simulink model "Modelo"  (R2018a)
settings: Solver=ode45  StartTime=0.0  StopTime=27  FixedStep=0.0001  MaxStep=1e-3
values from neighbouring files (symbols this model uses):
  d = 0.01    [setupSimulinkConstantes.m]
  erroInviavel_rotacao = pi    (= 3.14159265359)    [setupSimulinkConstantes.m]
  erroInviavel_translacao = 10    [setupSimulinkConstantes.m]
  J = 0.0015    [setupSimulinkConstantes.m]
  Kb = 0.4    [setupSimulinkConstantes.m]
  Kc = 4    [setupSimulinkConstantes.m]
  Kd = solucao(3)    [setupSimulinkSolucao.m]
  Ki = solucao(2)    [setupSimulinkSolucao.m]
  Kp = solucao(1)    [setupSimulinkSolucao.m]
  Kt = 0.4    [setupSimulinkConstantes.m]
  L = 0.1    [setupSimulinkConstantes.m]
  M = 0.25    [setupSimulinkConstantes.m]
  N = length(Xinit)    [Calcula_Delta_E.m]    (also in setupSimulinkConstantes.m = 30)
  Pista = 0    [ValidaResultado.m]    (also in fcusto_completa.m = i; fcusto_simplificada.m)
  R = 0.05    [setupSimulinkConstantes.m]
  Ra = 5e-3    (= 0.005)    [setupSimulinkConstantes.m]
  Va_med = 2.5    [setupSimulinkConstantes.m]
undefined symbols (not defined in the file or in its folder): sigbuilder_block
libraries: simulink x4
settings Model: SimulationMode=accelerator  Creator=root  LastModifiedBy=gabri
settings SolverCC: MaxConsecutiveZCs=100000  MaxConsecutiveMinStep=20
settings DataIOCC: ReturnWorkspaceOutputs=on
settings DebuggingCC: MaxConsecutiveZCsMsg=none  LibraryContextMissingDiagnostic=warning
settings SFSimCC: SimUseLocalCustomCode=on
settings RTWCC: RTWUseLocalCustomCode=on

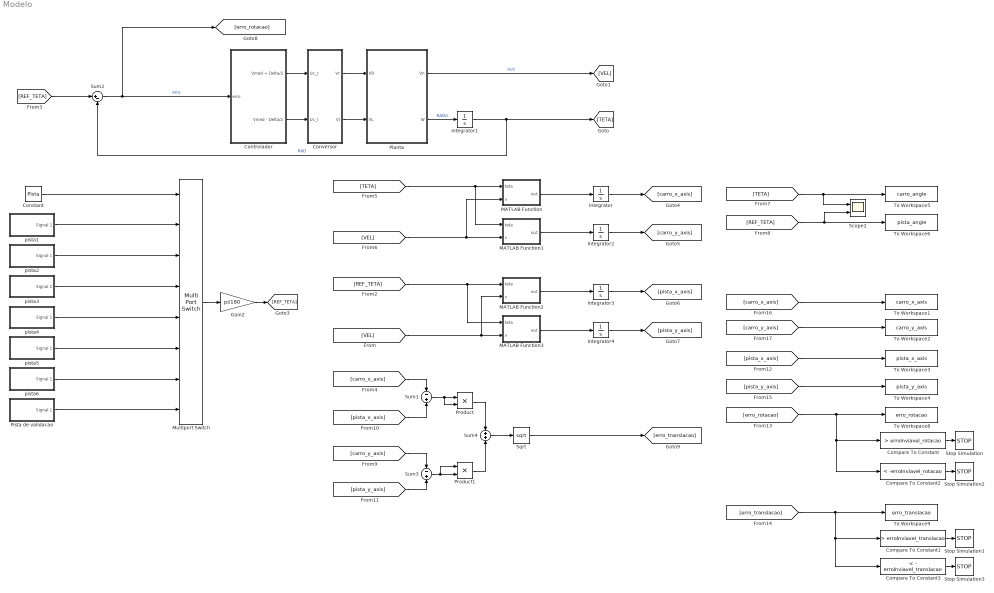
== system Modelo ==
  Compare To Constant : simulink/Logic and Bit Operations/Compare To Constant  relop=>  const=erroInviavel_rotacao  OutDataTypeStr=boolean
  Compare To Constant1 : simulink/Logic and Bit Operations/Compare To Constant  relop=>  const=erroInviavel_translacao  OutDataTypeStr=boolean
  Compare To Constant2 : simulink/Logic and Bit Operations/Compare To Constant  relop=<  const=-erroInviavel_rotacao  OutDataTypeStr=boolean
  Compare To Constant3 : simulink/Logic and Bit Operations/Compare To Constant  relop=<  const=- erroInviavel_translacao  OutDataTypeStr=boolean
  Constant : Constant  Value=Pista  VectorParams1D=off
  Controlador : Subsystem
  Conversor : Subsystem
  Gain2 : Gain  Gain=pi/180
  Integrator{,1..4} (5 alike) : Integrator
  MATLAB Function : MATLAB Function  TreatAsAtomicUnit=on
  MATLAB Function1 : MATLAB Function  TreatAsAtomicUnit=on
  MATLAB Function2 : MATLAB Function  TreatAsAtomicUnit=on
  MATLAB Function3 : MATLAB Function  TreatAsAtomicUnit=on
  Multiport Switch : MultiPortSwitch  Inputs=7  DiagnosticForDefault=None
  Pista de validacao : Subsystem  Tag=STV Subsys  LoadFcn=sigbuilder_block('load');  StartFcn=sigbuilder_block('start');  StopFcn=sigbuilder_block('stop');  ClipboardFcn=sigbuilder_block('clipboard');  mask(Sigbuilder block){tuvar=[0:10]}
      mask help: Simulink:masks:SigbuilderBlock_MD
      mask init:
      | if ~strcmp(get_param(bdroot(gcbh),'SimulationStatus'),'stopped') tuvar = sigbuilder_block('maskInit'); end
      settings: CopyFcn=sigbuilder_block('copy');  DeleteFcn=sigbuilder_block('delete');  ModelCloseFcn=sigbuilder_block('modelClose');  PreSaveFcn=sigbuilder_block('preSave');  PauseFcn=sigbuilder_block('pause');  ContinueFcn=sigbuilder_block('continue');  NameChangeFcn=sigbuilder_block('namechange');  OpenFcn=sigbuilder_block('open',[422.25 122.25 580.5 337.5 ]);  CloseFcn=sigbuilder_block('close');
      mask Display: plot(0, 0, 100, 100,[2, 2, 32, 32, 2], [68, 8, 8, 68, 68],[32, 2], [38, 38], [32, 19, 2],[53, 60, 44], [32, 17, 17, 2],[16, 16, 31, 31]);txt = getActiveGroup(gcbh);text(2, 100, txt,'verticalAlignment', 'top');
  Planta : Subsystem
  Product : Product
  Product1 : Product
  Scope2 : Scope  NumInputPorts=2
  Sqrt : Sqrt  SaturateOnIntegerOverflow=on
  Stop Simulation{,1..3} (4 alike) : Stop
  Sum1 : Sum  Inputs=-|+
  Sum2 : Sum  Inputs=|+-
  Sum3 : Sum  Inputs=-|+
  Sum4 : Sum  Inputs=+|+
  To Workspace1 : ToWorkspace  VariableName=carro_x_axis  SampleTime=-1
      settings: Save2DSignal=2-D array (concatenate along first dimension)
  To Workspace2 : ToWorkspace  VariableName=carro_y_axis  SampleTime=-1
      settings: Save2DSignal=2-D array (concatenate along first dimension)
  To Workspace3 : ToWorkspace  VariableName=pista_x_axis  SampleTime=-1
      settings: Save2DSignal=2-D array (concatenate along first dimension)
  To Workspace4 : ToWorkspace  VariableName=pista_y_axis  SampleTime=-1
      settings: Save2DSignal=2-D array (concatenate along first dimension)
  To Workspace5 : ToWorkspace  VariableName=carro_angle  SampleTime=-1
      settings: Save2DSignal=2-D array (concatenate along first dimension)
  To Workspace6 : ToWorkspace  VariableName=pista_angle  SampleTime=-1
      settings: Save2DSignal=2-D array (concatenate along first dimension)
  To Workspace8 : ToWorkspace  VariableName=erro_rotacao  SampleTime=-1
      settings: Save2DSignal=2-D array (concatenate along first dimension)
  To Workspace9 : ToWorkspace  VariableName=erro_translacao  SampleTime=-1
      settings: Save2DSignal=2-D array (concatenate along first dimension)
  pista1 : Subsystem  Tag=STV Subsys  LoadFcn=sigbuilder_block('load');  StartFcn=sigbuilder_block('start');  StopFcn=sigbuilder_block('stop');  ClipboardFcn=sigbuilder_block('clipboard');  mask(Sigbuilder block){tuvar=[0:10]}
      mask help: Simulink:masks:SigbuilderBlock_MD
      mask init:
      | if ~strcmp(get_param(bdroot(gcbh),'SimulationStatus'),'stopped') tuvar = sigbuilder_block('maskInit'); end
      settings: CopyFcn=sigbuilder_block('copy');  DeleteFcn=sigbuilder_block('delete');  ModelCloseFcn=sigbuilder_block('modelClose');  PreSaveFcn=sigbuilder_block('preSave');  PauseFcn=sigbuilder_block('pause');  ContinueFcn=sigbuilder_block('continue');  NameChangeFcn=sigbuilder_block('namechange');  OpenFcn=sigbuilder_block('open',[426 126 573 342.75 ]);  CloseFcn=sigbuilder_block('close');
      mask Display: plot(0, 0, 100, 100,[2, 2, 32, 32, 2], [68, 8, 8, 68, 68],[32, 2], [38, 38], [32, 19, 2],[53, 60, 44], [32, 17, 17, 2],[16, 16, 31, 31]);txt = getActiveGroup(gcbh);text(2, 100, txt,'verticalAlignment', 'top');
  pista2 : Subsystem  Tag=STV Subsys  LoadFcn=sigbuilder_block('load');  StartFcn=sigbuilder_block('start');  StopFcn=sigbuilder_block('stop');  ClipboardFcn=sigbuilder_block('clipboard');  mask(Sigbuilder block){tuvar=[0:10]}
      mask help: Simulink:masks:SigbuilderBlock_MD
      mask init:
      | if ~strcmp(get_param(bdroot(gcbh),'SimulationStatus'),'stopped') tuvar = sigbuilder_block('maskInit'); end
      settings: CopyFcn=sigbuilder_block('copy');  DeleteFcn=sigbuilder_block('delete');  ModelCloseFcn=sigbuilder_block('modelClose');  PreSaveFcn=sigbuilder_block('preSave');  PauseFcn=sigbuilder_block('pause');  ContinueFcn=sigbuilder_block('continue');  NameChangeFcn=sigbuilder_block('namechange');  OpenFcn=sigbuilder_block('open',[403.5 98.25 610.5 316.5 ]);  CloseFcn=sigbuilder_block('close');
      mask Display: plot(0, 0, 100, 100,[2, 2, 32, 32, 2], [68, 8, 8, 68, 68],[32, 2], [38, 38], [32, 19, 2],[53, 60, 44], [32, 17, 17, 2],[16, 16, 31, 31]);txt = getActiveGroup(gcbh);text(2, 100, txt,'verticalAlignment', 'top');
  pista3 : Subsystem  Tag=STV Subsys  LoadFcn=sigbuilder_block('load');  StartFcn=sigbuilder_block('start');  StopFcn=sigbuilder_block('stop');  ClipboardFcn=sigbuilder_block('clipboard');  mask(Sigbuilder block){tuvar=[0:10]}
      mask help: Simulink:masks:SigbuilderBlock_MD
      mask init:
      | if ~strcmp(get_param(bdroot(gcbh),'SimulationStatus'),'stopped') tuvar = sigbuilder_block('maskInit'); end
      settings: CopyFcn=sigbuilder_block('copy');  DeleteFcn=sigbuilder_block('delete');  ModelCloseFcn=sigbuilder_block('modelClose');  PreSaveFcn=sigbuilder_block('preSave');  PauseFcn=sigbuilder_block('pause');  ContinueFcn=sigbuilder_block('continue');  NameChangeFcn=sigbuilder_block('namechange');  OpenFcn=sigbuilder_block('open',[407.25 107.25 610.5 316.5 ]);  CloseFcn=sigbuilder_block('close');
      mask Display: plot(0, 0, 100, 100,[2, 2, 32, 32, 2], [68, 8, 8, 68, 68],[32, 2], [38, 38], [32, 19, 2],[53, 60, 44], [32, 17, 17, 2],[16, 16, 31, 31]);txt = getActiveGroup(gcbh);text(2, 100, txt,'verticalAlignment', 'top');
  pista4 : Subsystem  Tag=STV Subsys  LoadFcn=sigbuilder_block('load');  StartFcn=sigbuilder_block('start');  StopFcn=sigbuilder_block('stop');  ClipboardFcn=sigbuilder_block('clipboard');  mask(Sigbuilder block){tuvar=[0:10]}
      mask help: Simulink:masks:SigbuilderBlock_MD
      mask init:
      | if ~strcmp(get_param(bdroot(gcbh),'SimulationStatus'),'stopped') tuvar = sigbuilder_block('maskInit'); end
      settings: CopyFcn=sigbuilder_block('copy');  DeleteFcn=sigbuilder_block('delete');  ModelCloseFcn=sigbuilder_block('modelClose');  PreSaveFcn=sigbuilder_block('preSave');  PauseFcn=sigbuilder_block('pause');  ContinueFcn=sigbuilder_block('continue');  NameChangeFcn=sigbuilder_block('namechange');  OpenFcn=sigbuilder_block('open',[422.25 122.25 580.5 337.5 ]);  CloseFcn=sigbuilder_block('close');
      mask Display: plot(0, 0, 100, 100,[2, 2, 32, 32, 2], [68, 8, 8, 68, 68],[32, 2], [38, 38], [32, 19, 2],[53, 60, 44], [32, 17, 17, 2],[16, 16, 31, 31]);txt = getActiveGroup(gcbh);text(2, 100, txt,'verticalAlignment', 'top');
  pista5 : Subsystem  Tag=STV Subsys  LoadFcn=sigbuilder_block('load');  StartFcn=sigbuilder_block('start');  StopFcn=sigbuilder_block('stop');  ClipboardFcn=sigbuilder_block('clipboard');  mask(Sigbuilder block){tuvar=[0:10]}
      mask help: Simulink:masks:SigbuilderBlock_MD
      mask init:
      | if ~strcmp(get_param(bdroot(gcbh),'SimulationStatus'),'stopped') tuvar = sigbuilder_block('maskInit'); end
      settings: CopyFcn=sigbuilder_block('copy');  DeleteFcn=sigbuilder_block('delete');  ModelCloseFcn=sigbuilder_block('modelClose');  PreSaveFcn=sigbuilder_block('preSave');  PauseFcn=sigbuilder_block('pause');  ContinueFcn=sigbuilder_block('continue');  NameChangeFcn=sigbuilder_block('namechange');  OpenFcn=sigbuilder_block('open',[411 100.5 588 332.25 ]);  CloseFcn=sigbuilder_block('close');
      mask Display: plot(0, 0, 100, 100,[2, 2, 32, 32, 2], [68, 8, 8, 68, 68],[32, 2], [38, 38], [32, 19, 2],[53, 60, 44], [32, 17, 17, 2],[16, 16, 31, 31]);txt = getActiveGroup(gcbh);text(2, 100, txt,'verticalAlignment', 'top');
  pista6 : Subsystem  Tag=STV Subsys  LoadFcn=sigbuilder_block('load');  StartFcn=sigbuilder_block('start');  StopFcn=sigbuilder_block('stop');  ClipboardFcn=sigbuilder_block('clipboard');  mask(Sigbuilder block){tuvar=[0:10]}
      mask help: Simulink:masks:SigbuilderBlock_MD
      mask init:
      | if ~strcmp(get_param(bdroot(gcbh),'SimulationStatus'),'stopped') tuvar = sigbuilder_block('maskInit'); end
      settings: CopyFcn=sigbuilder_block('copy');  DeleteFcn=sigbuilder_block('delete');  ModelCloseFcn=sigbuilder_block('modelClose');  PreSaveFcn=sigbuilder_block('preSave');  PauseFcn=sigbuilder_block('pause');  ContinueFcn=sigbuilder_block('continue');  NameChangeFcn=sigbuilder_block('namechange');  OpenFcn=sigbuilder_block('open',[414.75 114.75 595.5 327 ]);  CloseFcn=sigbuilder_block('close');
      mask Display: plot(0, 0, 100, 100,[2, 2, 32, 32, 2], [68, 8, 8, 68, 68],[32, 2], [38, 38], [32, 19, 2],[53, 60, 44], [32, 17, 17, 2],[16, 16, 31, 31]);txt = getActiveGroup(gcbh);text(2, 100, txt,'verticalAlignment', 'top');
  wires:
  Sum2/1 -> Controlador/1(erro), [erro_rotacao]  "erro"
  Integrator1/1 -> Sum2/2, [TETA]  "RAD"
  Planta/1(Vn) -> [VEL]  "m/s"
  Controlador/1(Vmed + Delta/2) -> Conversor/1(Uc_r)
  Controlador/2(Vmed - Delta/2) -> Conversor/2(Uc_l)
  Conversor/1(Vr) -> Planta/1(VR)
  Conversor/2(Vl) -> Planta/2(VL)
  MATLAB Function2/1(out) -> Integrator3/1
  Integrator/1 -> [carro_x_axis]
  MATLAB Function1/1(out) -> Integrator2/1
  [VEL] -> MATLAB Function2/2(v), MATLAB Function3/2(v)
  [VEL] -> MATLAB Function/2(v), MATLAB Function1/2(v)
  MATLAB Function3/1(out) -> Integrator4/1
  [TETA] -> MATLAB Function1/1(teta), MATLAB Function/1(teta)
  MATLAB Function/1(out) -> Integrator/1
  Integrator2/1 -> [carro_y_axis]
  [REF_TETA] -> MATLAB Function3/1(teta), MATLAB Function2/1(teta)
  pista5/1(Signal 1) -> Multiport Switch/6
  pista6/1(Signal 1) -> Multiport Switch/7
  Pista de validacao/1(Signal 1) -> Multiport Switch/8
  pista2/1(Signal 1) -> Multiport Switch/3
  pista3/1(Signal 1) -> Multiport Switch/4
  pista4/1(Signal 1) -> Multiport Switch/5
  pista1/1(Signal 1) -> Multiport Switch/2
  Constant/1 -> Multiport Switch/1
  Multiport Switch/1 -> Gain2/1
  Gain2/1 -> [REF_TETA]
  [REF_TETA] -> Scope2/2, To Workspace6/1
  [TETA] -> Scope2/1, To Workspace5/1
  Planta/2(W) -> Integrator1/1  "RAD/s"
  Sum3/1 -> Product1/1, Product1/2
  Sum4/1 -> Sqrt/1
  [carro_y_axis] -> Sum3/1
  [pista_x_axis] -> Sum1/2
  [pista_y_axis] -> Sum3/2
  Sqrt/1 -> [erro_translacao]
  Product1/1 -> Sum4/2
  Product/1 -> Sum4/1
  Sum1/1 -> Product/2, Product/1
  [carro_x_axis] -> Sum1/1
  Integrator4/1 -> [pista_y_axis]
  Integrator3/1 -> [pista_x_axis]
  Compare To Constant1/1 -> Stop Simulation1/1
  Compare To Constant/1 -> Stop Simulation/1
  [pista_y_axis] -> To Workspace4/1
  [pista_x_axis] -> To Workspace3/1
  [carro_y_axis] -> To Workspace2/1
  [carro_x_axis] -> To Workspace1/1
  [REF_TETA] -> Sum2/1
  Compare To Constant2/1 -> Stop Simulation2/1
  [erro_rotacao] -> Compare To Constant2/1, Compare To Constant/1, To Workspace8/1
  [erro_translacao] -> Compare To Constant3/1, Compare To Constant1/1, To Workspace9/1
  Compare To Constant3/1 -> Stop Simulation3/1

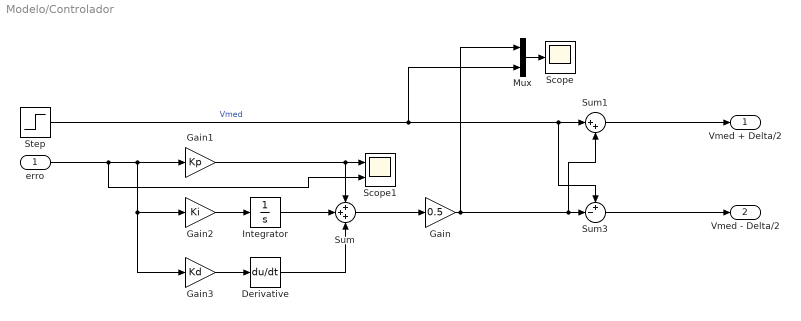
== system Modelo/Controlador ==
  erro : Inport
  Derivative : Derivative
  Gain : Gain  Gain=0.5
  Gain1 : Gain  Gain=Kp
  Gain2 : Gain  Gain=Ki
  Gain3 : Gain  Gain=Kd
  Integrator : Integrator
  Mux : Mux  Inputs=2
  Scope : Scope
  Scope1 : Scope  NumInputPorts=2
  Step : Step  Time=0  After=Va_med  SampleTime=0
  Sum : Sum  Inputs=+++
  Sum1 : Sum  Inputs=|++
  Sum3 : Sum  Inputs=+-|
  Vmed + Delta/2 : Outport
  Vmed - Delta/2 : Outport  Port=2
  wires:
  Sum3/1 -> Vmed - Delta/2/1
  Step/1 -> Mux/2, Sum1/1, Sum3/1  "Vmed"
  Sum1/1 -> Vmed + Delta/2/1
  Gain/1 -> Mux/1, Sum1/2, Sum3/2
  Mux/1 -> Scope/1
  erro/1 -> Scope1/2, Gain1/1, Gain3/1, Gain2/1
  Gain3/1 -> Derivative/1
  Gain2/1 -> Integrator/1
  Sum/1 -> Gain/1
  Integrator/1 -> Sum/2
  Derivative/1 -> Sum/3
  Gain1/1 -> Scope1/1, Sum/1

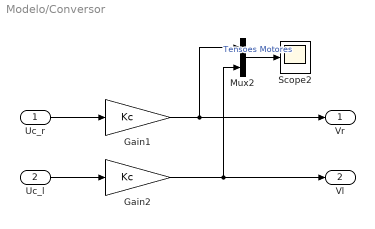
== system Modelo/Conversor ==
  Uc_r : Inport
  Uc_l : Inport  Port=2
  Gain1 : Gain  Gain=Kc
  Gain2 : Gain  Gain=Kc
  Mux2 : Mux  Inputs=2
  Scope2 : Scope
  Vr : Outport
  Vl : Outport  Port=2
  wires:
  Mux2/1 -> Scope2/1  "Tensoes Motores"
  Uc_l/1 -> Gain2/1
  Gain2/1 -> Vl/1, Mux2/2
  Uc_r/1 -> Gain1/1
  Gain1/1 -> Vr/1, Mux2/1

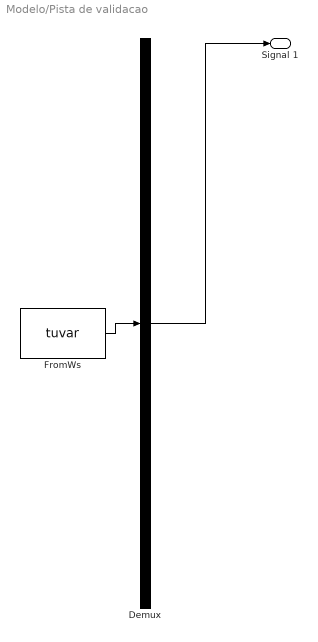
== system Modelo/Pista de validacao ==
  Demux : Demux  Tag=STV Demux  Outputs=1
  FromWs : FromWorkspace  Tag=STV FromWs  VariableName=tuvar  SampleTime=0
      SigBuilderData=|
      | common.afterFinalStr = 'Extrapolate'
      | common.sampleTime = 0
      | dataSet.timeRange = [0 27]
      | dataSet.name = 'Group 1'
      | sbobj.Groups.Name = 'Group 1'
      | sbobj.Groups.Signals.Name = 'Signal 1'
      | sbobj.Groups.Signals.XData = [0 1.392 1.643327 4.043327 4.294655 4.454655 4.705982 6.145982 6.39731 7.99731 8.499964 9.939964 10.693947 12.133947 12.510938 12.830938 12.956602 15.836602 16.087929 16.247929 16.62492 17.82492 18.201911 19.801911 20.053239 20.133239 20.258902 20.338902 22.97784 24.45784 24.583504 25.086159 25.588813 25.714477 25.874477 26.188636 27]
      | sbobj.Groups.Signals.YData = [0 0 -90 -90 -180 -180 -270 -270 -180 -180 -360 -360 -180 -180 -360 -360 -450 -450 -360 -360 -270 -270 -180 -180 -90 -90 0 0 -270 -270 -330 -210 -330 -270 -270 -360 -360]
      | sbobj.Groups.TimeRange = [0 27]
  Signal 1 : Outport  Tag=STV Outport
  wires:
  Demux/1 -> Signal 1/1
  FromWs/1 -> Demux/1

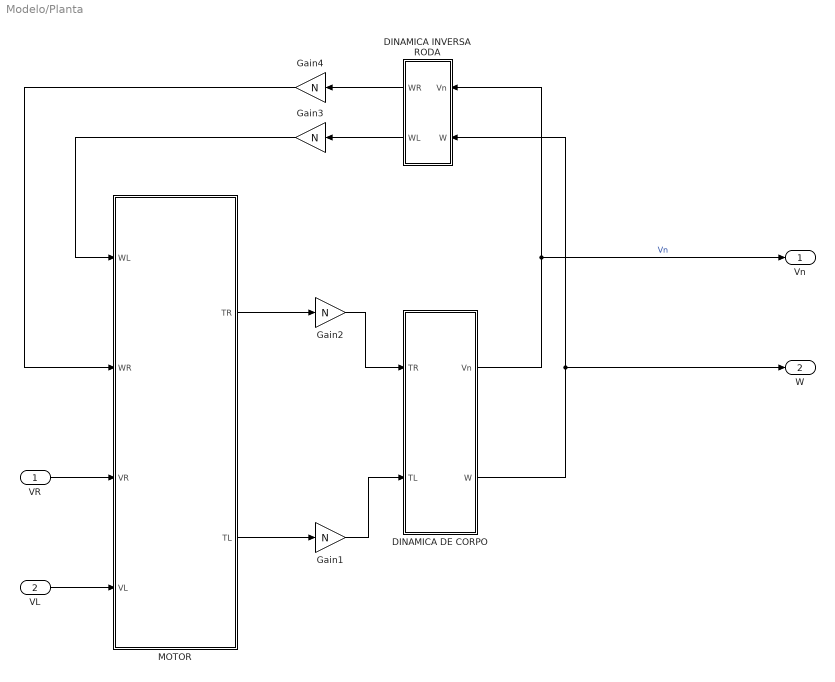
== system Modelo/Planta ==
  VR : Inport
  VL : Inport  Port=2
  DINAMICA DE CORPO : Subsystem
  DINAMICA INVERSA RODA : Subsystem
  Gain{1..4} (4 alike) : Gain  Gain=N
  MOTOR : Subsystem
  Vn : Outport
  W : Outport  Port=2
  wires:
  DINAMICA DE CORPO/1(Vn) -> DINAMICA INVERSA RODA/1(Vn), Vn/1  "Vn"
  DINAMICA INVERSA RODA/2(WL) -> Gain3/1
  DINAMICA INVERSA RODA/1(WR) -> Gain4/1
  MOTOR/1(TR) -> Gain2/1
  MOTOR/2(TL) -> Gain1/1
  VL/1 -> MOTOR/4(VL)
  DINAMICA DE CORPO/2(W) -> DINAMICA INVERSA RODA/2(W), W/1
  Gain2/1 -> DINAMICA DE CORPO/1(TR)
  Gain1/1 -> DINAMICA DE CORPO/2(TL)
  Gain3/1 -> MOTOR/1(WL)
  Gain4/1 -> MOTOR/2(WR)
  VR/1 -> MOTOR/3(VR)

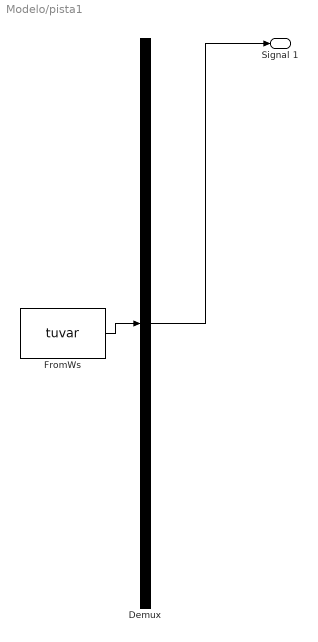
== system Modelo/pista1 ==
  Demux : Demux  Tag=STV Demux  Outputs=1
  FromWs : FromWorkspace  Tag=STV FromWs  VariableName=tuvar  SampleTime=0
      SigBuilderData=|
      | common.afterFinalStr = 'Extrapolate'
      | common.sampleTime = 0
      | dataSet.timeRange = [0 10]
      | dataSet.name = 'Group 1'
      | sbobj.Groups.Name = 'Group 1'
      | sbobj.Groups.Signals.Name = 'Signal 1'
      | sbobj.Groups.Signals.XData = [0 1.392 1.643327 4.043327 4.294655 4.454655 4.705982 6.145982 6.39731 7.99731 8.499964 9.939964 10]
      | sbobj.Groups.Signals.YData = [0 0 -90 -90 -180 -180 -270 -270 -180 -180 -360 -360 -345.667475261]
  Signal 1 : Outport  Tag=STV Outport
  wires:
  Demux/1 -> Signal 1/1
  FromWs/1 -> Demux/1

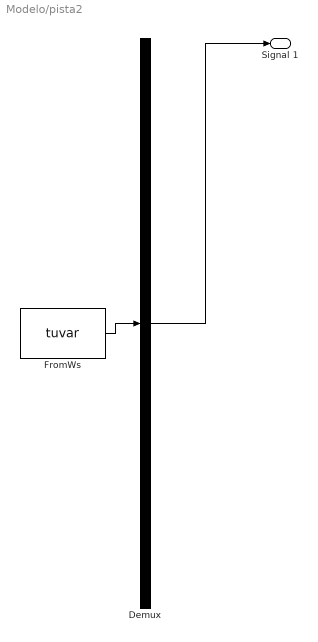
== system Modelo/pista2 ==
  Demux : Demux  Tag=STV Demux  Outputs=1
  FromWs : FromWorkspace  Tag=STV FromWs  VariableName=tuvar  SampleTime=0
      SigBuilderData=|
      | common.afterFinalStr = 'Extrapolate'
      | common.sampleTime = 0
      | dataSet.timeRange = [0 27]
      | dataSet.name = 'Group 1'
      | sbobj.Groups.Name = 'Group 1'
      | sbobj.Groups.Signals.Name = 'Signal 1'
      | sbobj.Groups.Signals.XData = [0 1.884956 3.769911 4.900885 5.466371 27]
      | sbobj.Groups.Signals.YData = [270 270 0 -270 -540 -540]
      | sbobj.Groups.TimeRange = [0 27]
  Signal 1 : Outport  Tag=STV Outport
  wires:
  Demux/1 -> Signal 1/1
  FromWs/1 -> Demux/1

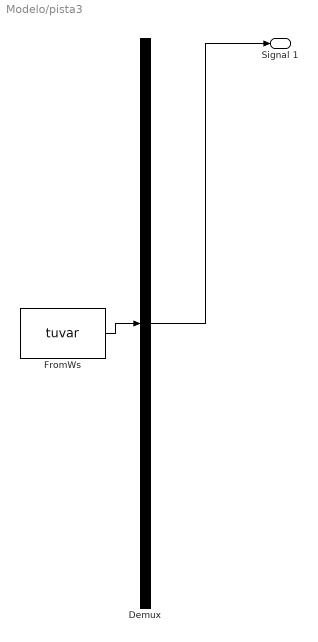
== system Modelo/pista3 ==
  Demux : Demux  Tag=STV Demux  Outputs=1
  FromWs : FromWorkspace  Tag=STV FromWs  VariableName=tuvar  SampleTime=0
      SigBuilderData=|
      | common.afterFinalStr = 'Extrapolate'
      | common.sampleTime = 0
      | dataSet.timeRange = [0 27]
      | dataSet.name = 'Group 1'
      | sbobj.Groups.Name = 'Group 1'
      | sbobj.Groups.Signals.Name = 'Signal 1'
      | sbobj.Groups.Signals.XData = [0 1.656637 2.913274 27]
      | sbobj.Groups.Signals.YData = [180 180 360 360]
      | sbobj.Groups.TimeRange = [0 27]
  Signal 1 : Outport  Tag=STV Outport
  wires:
  Demux/1 -> Signal 1/1
  FromWs/1 -> Demux/1

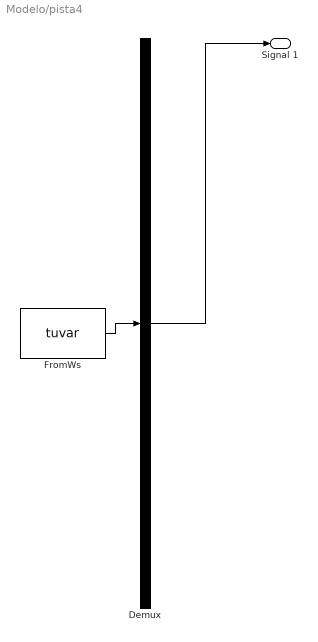
== system Modelo/pista4 ==
  Demux : Demux  Tag=STV Demux  Outputs=1
  FromWs : FromWorkspace  Tag=STV FromWs  VariableName=tuvar  SampleTime=0
      SigBuilderData=|
      | common.afterFinalStr = 'Extrapolate'
      | common.sampleTime = 0
      | dataSet.timeRange = [0 27]
      | dataSet.name = 'Group 1'
      | sbobj.Groups.Name = 'Group 1'
      | sbobj.Groups.Signals.Name = 'Signal 1'
      | sbobj.Groups.Signals.XData = [0 0.24 0.302832 0.554159 0.805487 1.056814 1.308142 1.559469 1.810796 2.062124 2.313451 2.564779 2.816106 3.067433 3.318761 3.570088 3.821416 4.072743 4.32407 4.575398 4.826725 5.078053 5.32938 5.580708 5.832035 6.083362 6.33469 6.586017 6.837345 7.088672 7.339999 7.591327 7.654159 7.894159 8.082654 27]
      | sbobj.Groups.Signals.YData = [0 0 -30 -150 -30 -150 -30 -150 -30 -150 -30 -150 -30 -150 -30 -150 -30 -150 -30 -150 -30 -150 -30 -150 -30 -150 -30 -150 -30 -150 -30 -150 -180 -180 -270 -270]
      | sbobj.Groups.TimeRange = [0 27]
  Signal 1 : Outport  Tag=STV Outport
  wires:
  Demux/1 -> Signal 1/1
  FromWs/1 -> Demux/1

== system Modelo/pista5 ==
  Demux : Demux  Tag=STV Demux  Outputs=1
  FromWs : FromWorkspace  Tag=STV FromWs  VariableName=tuvar  SampleTime=0
      SigBuilderData=|
      | common.afterFinalStr = 'Extrapolate'
      | common.sampleTime = 0
      | dataSet.timeRange = [0 27]
      | dataSet.name = 'Group 1'
      | sbobj.Groups.Name = 'Group 1'
      | sbobj.Groups.Signals.Name = 'Signal 1'
      | sbobj.Groups.Signals.XData = [0 0.24 0.616991 0.736991 1.113982 1.233982 1.610973 1.730973 2.107964 2.227964 2.604956 2.724956 3.101947 3.221947 3.598938 3.718938 4.095929 4.215929 4.59292 4.71292 5.089911 5.209911 5.586902 5.706902 6.083893 6.203893 6.580885 6.700885 7.077876 7.197876 7.574867 7.694867 8.071858 8.191858 8.568849 8.688849 9.06584 9.18584 9.562831 9.922831 10.111327 27]
      | sbobj.Groups.Signals.YData = [0 0 -180 -180 0 0 -180 -180 0 0 -180 -180 0 0 -180 -180 0 0 -180 -180 0 0 -180 -180 0 0 -180 -180 0 0 -180 -180 0 0 -180 -180 0 0 -180 -180 -270 -270]
      | sbobj.Groups.TimeRange = [0 27]
  Signal 1 : Outport  Tag=STV Outport
  wires:
  Demux/1 -> Signal 1/1
  FromWs/1 -> Demux/1

== system Modelo/pista6 ==
  Demux : Demux  Tag=STV Demux  Outputs=1
  FromWs : FromWorkspace  Tag=STV FromWs  VariableName=tuvar  SampleTime=0
      SigBuilderData=|
      | common.afterFinalStr = 'Extrapolate'
      | common.sampleTime = 0
      | dataSet.timeRange = [0 4.5]
      | dataSet.name = 'Group 1'
      | sbobj.Groups.Name = 'Group 1'
      | sbobj.Groups.Signals.Name = 'Signal 1'
      | sbobj.Groups.Signals.XData = [0 0.48 0.49885 0.97885 0.997699 1.477699 1.496549 1.976549 1.995398 2.475398 2.494248 2.974248 2.993097 3.473097 3.491947 3.971947 3.990796 4.5]
      | sbobj.Groups.Signals.YData = [0 0 45 45 90 90 135 135 180 180 225 225 270 270 315 315 360 360]
      | sbobj.Groups.TimeRange = [0 4.5]
  Signal 1 : Outport  Tag=STV Outport
  wires:
  Demux/1 -> Signal 1/1
  FromWs/1 -> Demux/1

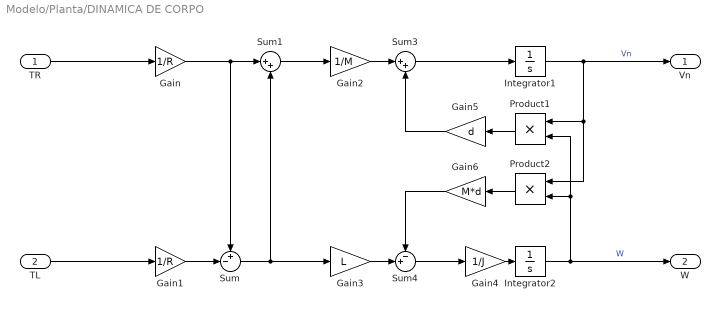
== system Modelo/Planta/DINAMICA DE CORPO ==
  TR : Inport
  TL : Inport  Port=2
  Gain : Gain  Gain=1/R
  Gain1 : Gain  Gain=1/R
  Gain2 : Gain  Gain=1/M
  Gain3 : Gain  Gain=L
  Gain4 : Gain  Gain=1/J
  Gain5 : Gain  Gain=d
  Gain6 : Gain  Gain=M*d
  Integrator1 : Integrator
  Integrator2 : Integrator
  Product1 : Product
  Product2 : Product
  Sum : Sum  Inputs=+-|
  Sum1 : Sum  Inputs=|++
  Sum3 : Sum  Inputs=|++
  Sum4 : Sum  Inputs=-+|
  Vn : Outport
  W : Outport  Port=2
  wires:
  Sum3/1 -> Integrator1/1
  Gain5/1 -> Sum3/2
  Product1/1 -> Gain5/1
  Gain3/1 -> Sum4/2
  Gain1/1 -> Sum/2
  Sum/1 -> Sum1/2, Gain3/1
  Product2/1 -> Gain6/1
  Gain2/1 -> Sum3/1
  Integrator1/1 -> Vn/1, Product2/1, Product1/1  "Vn"
  Sum1/1 -> Gain2/1
  TR/1 -> Gain/1
  TL/1 -> Gain1/1
  Gain4/1 -> Integrator2/1
  Sum4/1 -> Gain4/1
  Gain6/1 -> Sum4/1
  Integrator2/1 -> W/1, Product1/2, Product2/2  "W"
  Gain/1 -> Sum1/1, Sum/1

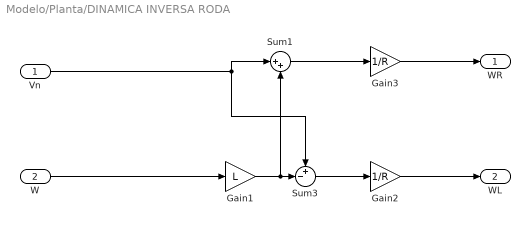
== system Modelo/Planta/DINAMICA INVERSA RODA ==
  Vn : Inport
  W : Inport  Port=2
  Gain1 : Gain  Gain=L
  Gain2 : Gain  Gain=1/R
  Gain3 : Gain  Gain=1/R
  Sum1 : Sum  Inputs=|++
  Sum3 : Sum  Inputs=+-|
  WR : Outport
  WL : Outport  Port=2
  wires:
  Gain3/1 -> WR/1
  W/1 -> Gain1/1
  Vn/1 -> Sum1/1, Sum3/1
  Sum3/1 -> Gain2/1
  Gain2/1 -> WL/1
  Sum1/1 -> Gain3/1
  Gain1/1 -> Sum1/2, Sum3/2

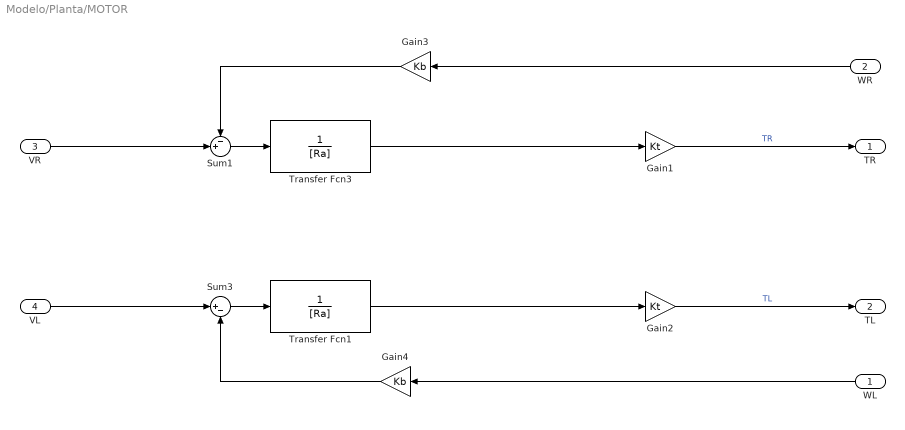
== system Modelo/Planta/MOTOR ==
  WL : Inport
  WR : Inport  Port=2
  VR : Inport  Port=3
  VL : Inport  Port=4
  Gain1 : Gain  Gain=Kt
  Gain2 : Gain  Gain=Kt
  Gain3 : Gain  Gain=Kb
  Gain4 : Gain  Gain=Kb
  Sum1 : Sum  Inputs=-+|
  Sum3 : Sum  Inputs=|+-
  Transfer Fcn1 : TransferFcn  Denominator=[Ra]
  Transfer Fcn3 : TransferFcn  Denominator=[Ra]
  TR : Outport
  TL : Outport  Port=2
  wires:
  Sum1/1 -> Transfer Fcn3/1
  Gain4/1 -> Sum3/2
  Sum3/1 -> Transfer Fcn1/1
  Gain1/1 -> TR/1  "TR"
  WR/1 -> Gain3/1
  Gain3/1 -> Sum1/1
  Gain2/1 -> TL/1  "TL"
  WL/1 -> Gain4/1
  VR/1 -> Sum1/2
  VL/1 -> Sum3/1
  Transfer Fcn3/1 -> Gain1/1
  Transfer Fcn1/1 -> Gain2/1

== matlab function Modelo/MATLAB Function1 ==
  data: teta input; out output; v input
function out = fcn_y(teta, v)
 
out = cos(teta)*v;

== matlab function Modelo/MATLAB Function ==
  data: teta input; out output; v input
function out = fcn_x(teta, v)
 
out = sin(teta)*v;

== matlab function Modelo/MATLAB Function2 ==
  data: teta input; out output; v input
function out = fcn_x(teta, v)
 
out = sin(teta)*v;

== matlab function Modelo/MATLAB Function3 ==
  data: teta input; out output; v input
function out = fcn_y(teta, v)
 
out = cos(teta)*v;
